simulink model "Drone_Model_Initial"  (R2024b)
settings: Solver=VariableStepAuto  StartTime=0.0  StopTime=22.5  MaxStep=1e-4  RelTol=1e-3
values from neighbouring files (symbols this model uses):
  Kd_angle = 2.6    [MainScript.m]
  Kd_angle_psi = 2.6    [MainScript.m]
  Kd_dist = 1.05    [MainScript.m]
  Kd_z = 4.4    [MainScript.m]
  Ki_angle = 0.5    [MainScript.m]
  Ki_angle_psi = 0.5    [MainScript.m]
  Ki_dist = 0    [MainScript.m]
  Ki_z = 0.1    [MainScript.m]
  Kp_angle = 2.95    [MainScript.m]
  Kp_angle_psi = 2.95    [MainScript.m]
  Kp_dist = 1    [MainScript.m]
  Kp_z = 2    [MainScript.m]
  p1 = (Iyy - Izz) / Ixx    [linearizeSystem.m]
  p3 = (Ixx - Iyy) / Iyy    [linearizeSystem.m]
  p4 = 1 / Iyy    [linearizeSystem.m]
  p6 = 1 / Izz    [linearizeSystem.m]
undefined symbols (not defined in the file or in its folder): g, K, m, Omega_sq_2_U, p7, phi_0, phi_dot_0, phi_limit, psi_0, psi_dot_0, th_0, th_dot_0, theta_limit, U_Sq_max, U_to_Omega_sq, x_0, x_dot_0, y_0, y_dot_0, z_0, z_dot_0
libraries: slpidlib x6, simulink x1
settings Model: Creator=jkord  LastModifiedBy=steli

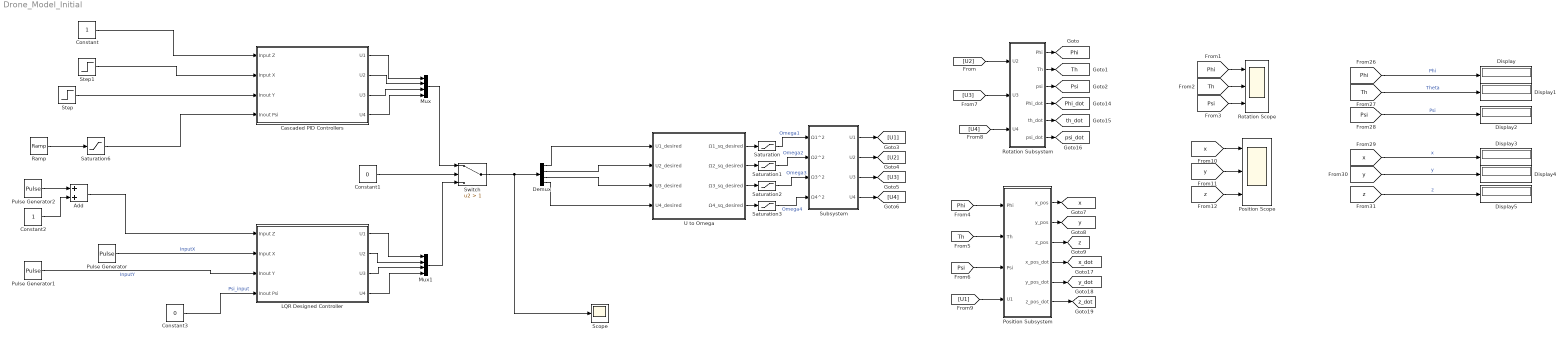
== system Drone_Model_Initial ==
  Add : Sum
  Cascaded PID Controllers : Subsystem
  Constant : Constant
  Constant1 : Constant  Value=0
  Constant2 : Constant
  Constant3 : Constant  Value=0
  Demux : Demux
  Display{,1..5} (6 alike) : Display
  LQR Designed Controller : Subsystem
  Mux : Mux
  Mux1 : Mux
  Position Subsystem : Subsystem
  Position Scope : Scope  NumInputPorts=3
  Pulse Generator : DiscretePulseGenerator  PulseType=Time based  Period=10  PulseWidth=50  PhaseDelay=2.5
  Pulse Generator1 : DiscretePulseGenerator  PulseType=Time based  Period=20  PulseWidth=50  PhaseDelay=10
  Pulse Generator2 : DiscretePulseGenerator  PulseType=Time based  Period=20  PulseWidth=50  PhaseDelay=5
  Ramp : simulink/Sources/Ramp  slope=0.01  start=2  InitialOutput=0
  Rotation Subsystem : Subsystem
  Rotation Scope : Scope  NumInputPorts=3
  Saturation{,1..3} (4 alike) : Saturate  UpperLimit=U_Sq_max  LowerLimit=0
  Saturation6 : Saturate  UpperLimit=0.2  LowerLimit=0
  Scope : Scope
  Step : Step  Time=5  SampleTime=0
  Step1 : Step  Time=2  SampleTime=0
  Subsystem : Subsystem
  Switch : Switch  Criteria=u2 > Threshold  Threshold=1  SaturateOnIntegerOverflow=off  InputSameDT=off
  U to Omega : Subsystem
  tag scope: Phi=global, Phi_dot=global, Psi=global, Th=global, psi_dot=global, th_dot=global, x=global, x_dot=global, y=global, y_dot=global, z=global, z_dot=global
  wires:
  [Th] -> Position Subsystem/2(Th)
  [U3] -> Rotation Subsystem/2(U3)
  Rotation Subsystem/3(psi) -> [Psi]
  [U4] -> Rotation Subsystem/3(U4)
  Rotation Subsystem/1(Phi) -> [Phi]
  Rotation Subsystem/2(Th) -> [Th]
  Position Subsystem/6(z_pos_dot) -> [z_dot]
  [Phi] -> Position Subsystem/1(Phi)
  Rotation Subsystem/4(Phi_dot) -> [Phi_dot]
  Rotation Subsystem/5(th_dot) -> [th_dot]
  Position Subsystem/4(x_pos_dot) -> [x_dot]
  [Psi] -> Position Subsystem/3(Psi)
  Position Subsystem/5(y_pos_dot) -> [y_dot]
  Position Subsystem/1(x_pos) -> [x]
  [U1] -> Position Subsystem/4(U1)
  Position Subsystem/3(z_pos) -> [z]
  Position Subsystem/2(y_pos) -> [y]
  [U2] -> Rotation Subsystem/1(U2)
  U to Omega/1(Ω1_sq_desired) -> Saturation/1
  Saturation3/1 -> Subsystem/4(Ω4^2)  "Omega4"
  U to Omega/3(Ω3_sq_desired) -> Saturation2/1
  U to Omega/2(Ω2_sq_desired) -> Saturation1/1
  Saturation2/1 -> Subsystem/3(Ω3^2)  "Omega3"
  Saturation1/1 -> Subsystem/2(Ω2^2)  "Omega2"
  U to Omega/4(Ω4_sq_desired) -> Saturation3/1
  Subsystem/4(U4) -> [U4]
  Saturation/1 -> Subsystem/1(Ω1^2)  "Omega1"
  Subsystem/2(U2) -> [U2]
  Subsystem/3(U3) -> [U3]
  Subsystem/1(U1) -> [U1]
  [Psi] -> Rotation Scope/3
  [z] -> Display5/1  "z"
  [Psi] -> Display2/1  "Psi"
  [Th] -> Rotation Scope/2
  [Th] -> Display1/1  "Theta"
  [y] -> Position Scope/2
  [Phi] -> Rotation Scope/1
  [z] -> Position Scope/3
  [Phi] -> Display/1  "Phi"
  [x] -> Display3/1  "x"
  [y] -> Display4/1  "y"
  [x] -> Position Scope/1
  Ramp/1 -> Saturation6/1
  Constant/1 -> Cascaded PID Controllers/1(Input Z)
  Step1/1 -> Cascaded PID Controllers/2(Input X)
  Step/1 -> Cascaded PID Controllers/3(Inout Y)
  Saturation6/1 -> Cascaded PID Controllers/4(Inout Psi)
  Cascaded PID Controllers/1(U1) -> Mux/1
  Cascaded PID Controllers/2(U2) -> Mux/2
  Cascaded PID Controllers/3(U3) -> Mux/3
  Cascaded PID Controllers/4(U4) -> Mux/4
  Mux/1 -> Switch/1
  Switch/1 -> Scope/1, Demux/1
  Demux/1 -> U to Omega/1(U1_desired)
  Demux/2 -> U to Omega/2(U2_desired)
  Demux/3 -> U to Omega/3(U3_desired)
  Demux/4 -> U to Omega/4(U4_desired)
  Constant1/1 -> Switch/2
  LQR Designed Controller/2(U2) -> Mux1/2
  LQR Designed Controller/1(U1) -> Mux1/1
  LQR Designed Controller/3(U3) -> Mux1/3
  LQR Designed Controller/4(U4) -> Mux1/4
  Mux1/1 -> Switch/3
  Rotation Subsystem/6(psi_dot) -> [psi_dot]
  Pulse Generator/1 -> LQR Designed Controller/2(Input X)  "InputX"
  Pulse Generator1/1 -> LQR Designed Controller/3(Inout Y)  "InputY"
  Pulse Generator2/1 -> Add/1
  Constant2/1 -> Add/2
  Add/1 -> LQR Designed Controller/1(Input Z)
  Constant3/1 -> LQR Designed Controller/4(Inout Psi)  "Psi_input"

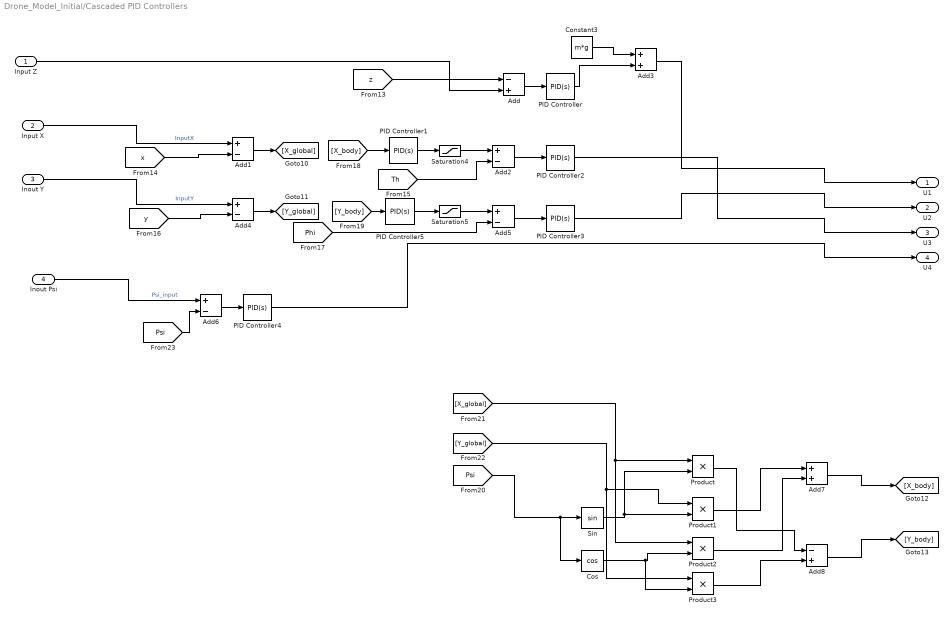
== system Drone_Model_Initial/Cascaded PID Controllers ==
  Input Z : Inport
  Input X : Inport  Port=2
  Inout Y : Inport  Port=3
  Inout Psi : Inport  Port=4
  Add : Sum  Inputs=-+
  Add{1..2,4..6} (5 alike) : Sum  Inputs=+-
  Add3 : Sum
  Add7 : Sum
  Add8 : Sum  Inputs=-+
  Constant3 : Constant  Value=m*g
  Cos : Trigonometry  Operator=cos
  PID Controller : slpidlib/PID Controller  Controller=PID  Form=Parallel  TimeDomain=Continuous-time  UseExternalTs=off  SampleTime=-1  IntegratorMethod=Forward Euler  FilterMethod=Forward Euler  ControllerParametersSource=internal  P=Kp_z  I=Ki_z  UseKiTs=off  D=Kd_z  UseExternalDerivativeSource=off  N=100  UseFilter=on  TunerSelectOption=Transfer Function Based (PID Tuner App)  InitialConditionSource=internal  InitialConditionForIntegrator=0  InitialConditionForFilter=0  DifferentiatorICPrevScaledInput=0  ExternalReset=none  TrackingMode=off  Kt=1  LimitOutput=off  SatLimitsSource=internal  UpperSaturationLimit=inf  LowerSaturationLimit=-inf  LinearizeAsGain=on  AntiWindupMode=none  Kb=1  LimitIntegrator=off  UpperIntegratorSaturationLimit=inf  LowerIntegratorSaturationLimit=-inf  POutMin=[]  POutMax=[]  IOutMin=[]  IOutMax=[]  DOutMin=[]  DOutMax=[]  NOutMin=[]  NOutMax=[]  SumOutMin=[]  SumOutMax=[]  SaturationOutMin=[]  SaturationOutMax=[]  PParamMin=[]  PParamMax=[]  IParamMin=[]  IParamMax=[]  DParamMin=[]  DParamMax=[]  NParamMin=[]  NParamMax=[]  KbParamMin=[]  KbParamMax=[]  KtParamMin=[]  KtParamMax=[]  KbOutMin=[]  KbOutMax=[]  KtOutMin=[]  KtOutMax=[]  IntegratorOutMin=[]  IntegratorOutMax=[]  FilterOutMin=[]  FilterOutMax=[]  SumI1OutMin=[]  SumI1OutMax=[]  SumI2OutMin=[]  SumI2OutMax=[]  SumI3OutMin=[]  SumI3OutMax=[]  SumI4OutMin=[]  SumI4OutMax=[]  SumDOutMin=[]  SumDOutMax=[]  DifferentiatorOutMin=[]  DifferentiatorOutMax=[]  FilterDiffOutCoefMin=[]  FilterDiffOutCoefMax=[]  ReciprocalOutMin=[]  ReciprocalOutMax=[]  SumDenOutMin=[]  SumDenOutMax=[]  SumNumOutMin=[]  SumNumOutMax=[]  DivideOutMin=[]  DivideOutMax=[]  UdiffTsProdOutMin=[]  UdiffTsProdOutMax=[]  NTsProdOutMin=[]  NTsProdOutMax=[]  UintegralTsProdOutMin=[]  UintegralTsProdOutMax=[]  UngainTsProdOutMin=[]  UngainTsProdOutMax=[]  ClampingZeroOutDataTypeStr=Inherit: Inherit via back propagation  ClampingZeroOutMin=[]  ClampingZeroOutMax=[]  FilterDenConstantOutDataTypeStr=Inherit: Inherit via back propagation  FilterDenConstantOutMin=[]  FilterDenConstantOutMax=[]  PCopyOutDataTypeStr=Inherit: Inherit via back propagation  PCopyOutMin=[]  PCopyOutMax=[]  NCopyOutDataTypeStr=Inherit: Inherit via back propagation  NCopyOutMin=[]  NCopyOutMax=[]  IntegratorContinuousStateAttributes=''  IntegratorStateMustResolveToSignalObject=off  IntegratorRTWStateStorageClass=Auto  FilterContinuousStateAttributes=''  FilterStateMustResolveToSignalObject=off  FilterRTWStateStorageClass=Auto  ParallelPVariant=InternalParameters  IdealPVariant=Disabled  IVariant=InternalParameters  DVariant=InternalParameters  IntegratorVariant=Continuous  SatVariant=Disabled  AWVariant=Passthrough  PCopyVariant=Disabled  TRVariant=Disabled  FdbkBlocksVariant=Forward  IdealPFdbkVariant=Disabled  SatFdbkVariant=Disabled  DerivativeFilterVariant=ContFilter  NVariant=InternalParameters  NCopyVariant=Disabled  FilterICVariant=InternalICsFilter  IntegratorICVariant=InternalICs  ExternalResetVariant=Disabled  TRSumVariant=Passthrough  SumFdbkVariant=Disabled  SumVariant=Sum_PID  TsampFilterVariant=InternalTs  TsampNgainVariant=Passthrough  TsampIntegralVariant=Disabled_SignalSpec  ExternalSaturationOutDataTypeStr=Inherit: Same as second input  DerivativeSourceVariant=ErrorSignal  PreIntVariant=InternalPreInt
  PID Controller1 : slpidlib/PID Controller  Controller=PID  Form=Parallel  TimeDomain=Continuous-time  UseExternalTs=off  SampleTime=-1  IntegratorMethod=Forward Euler  FilterMethod=Forward Euler  ControllerParametersSource=internal  P=Kp_dist  I=Ki_dist  UseKiTs=off  D=Kd_dist  UseExternalDerivativeSource=off  N=100  UseFilter=on  TunerSelectOption=Transfer Function Based (PID Tuner App)  InitialConditionSource=internal  InitialConditionForIntegrator=0  InitialConditionForFilter=0  DifferentiatorICPrevScaledInput=0  ExternalReset=none  TrackingMode=off  Kt=1  LimitOutput=off  SatLimitsSource=internal  UpperSaturationLimit=inf  LowerSaturationLimit=-inf  LinearizeAsGain=on  AntiWindupMode=none  Kb=1  LimitIntegrator=off  UpperIntegratorSaturationLimit=inf  LowerIntegratorSaturationLimit=-inf  POutMin=[]  POutMax=[]  IOutMin=[]  IOutMax=[]  DOutMin=[]  DOutMax=[]  NOutMin=[]  NOutMax=[]  SumOutMin=[]  SumOutMax=[]  SaturationOutMin=[]  SaturationOutMax=[]  PParamMin=[]  PParamMax=[]  IParamMin=[]  IParamMax=[]  DParamMin=[]  DParamMax=[]  NParamMin=[]  NParamMax=[]  KbParamMin=[]  KbParamMax=[]  KtParamMin=[]  KtParamMax=[]  KbOutMin=[]  KbOutMax=[]  KtOutMin=[]  KtOutMax=[]  IntegratorOutMin=[]  IntegratorOutMax=[]  FilterOutMin=[]  FilterOutMax=[]  SumI1OutMin=[]  SumI1OutMax=[]  SumI2OutMin=[]  SumI2OutMax=[]  SumI3OutMin=[]  SumI3OutMax=[]  SumI4OutMin=[]  SumI4OutMax=[]  SumDOutMin=[]  SumDOutMax=[]  DifferentiatorOutMin=[]  DifferentiatorOutMax=[]  FilterDiffOutCoefMin=[]  FilterDiffOutCoefMax=[]  ReciprocalOutMin=[]  ReciprocalOutMax=[]  SumDenOutMin=[]  SumDenOutMax=[]  SumNumOutMin=[]  SumNumOutMax=[]  DivideOutMin=[]  DivideOutMax=[]  UdiffTsProdOutMin=[]  UdiffTsProdOutMax=[]  NTsProdOutMin=[]  NTsProdOutMax=[]  UintegralTsProdOutMin=[]  UintegralTsProdOutMax=[]  UngainTsProdOutMin=[]  UngainTsProdOutMax=[]  ClampingZeroOutDataTypeStr=Inherit: Inherit via back propagation  ClampingZeroOutMin=[]  ClampingZeroOutMax=[]  FilterDenConstantOutDataTypeStr=Inherit: Inherit via back propagation  FilterDenConstantOutMin=[]  FilterDenConstantOutMax=[]  PCopyOutDataTypeStr=Inherit: Inherit via back propagation  PCopyOutMin=[]  PCopyOutMax=[]  NCopyOutDataTypeStr=Inherit: Inherit via back propagation  NCopyOutMin=[]  NCopyOutMax=[]  IntegratorContinuousStateAttributes=''  IntegratorStateMustResolveToSignalObject=off  IntegratorRTWStateStorageClass=Auto  FilterContinuousStateAttributes=''  FilterStateMustResolveToSignalObject=off  FilterRTWStateStorageClass=Auto  ParallelPVariant=InternalParameters  IdealPVariant=Disabled  IVariant=InternalParameters  DVariant=InternalParameters  IntegratorVariant=Continuous  SatVariant=Disabled  AWVariant=Passthrough  PCopyVariant=Disabled  TRVariant=Disabled  FdbkBlocksVariant=Forward  IdealPFdbkVariant=Disabled  SatFdbkVariant=Disabled  DerivativeFilterVariant=ContFilter  NVariant=InternalParameters  NCopyVariant=Disabled  FilterICVariant=InternalICsFilter  IntegratorICVariant=InternalICs  ExternalResetVariant=Disabled  TRSumVariant=Passthrough  SumFdbkVariant=Disabled  SumVariant=Sum_PID  TsampFilterVariant=InternalTs  TsampNgainVariant=Passthrough  TsampIntegralVariant=Disabled_SignalSpec  ExternalSaturationOutDataTypeStr=Inherit: Same as second input  DerivativeSourceVariant=ErrorSignal  PreIntVariant=InternalPreInt
  PID Controller2 : slpidlib/PID Controller  Controller=PID  Form=Parallel  TimeDomain=Continuous-time  UseExternalTs=off  SampleTime=-1  IntegratorMethod=Forward Euler  FilterMethod=Forward Euler  ControllerParametersSource=internal  P=Kp_angle  I=Ki_angle  UseKiTs=off  D=Kd_angle  UseExternalDerivativeSource=off  N=100  UseFilter=on  TunerSelectOption=Transfer Function Based (PID Tuner App)  InitialConditionSource=internal  InitialConditionForIntegrator=0  InitialConditionForFilter=0  DifferentiatorICPrevScaledInput=0  ExternalReset=none  TrackingMode=off  Kt=1  LimitOutput=off  SatLimitsSource=internal  UpperSaturationLimit=inf  LowerSaturationLimit=-inf  LinearizeAsGain=on  AntiWindupMode=none  Kb=1  LimitIntegrator=off  UpperIntegratorSaturationLimit=inf  LowerIntegratorSaturationLimit=-inf  POutMin=[]  POutMax=[]  IOutMin=[]  IOutMax=[]  DOutMin=[]  DOutMax=[]  NOutMin=[]  NOutMax=[]  SumOutMin=[]  SumOutMax=[]  SaturationOutMin=[]  SaturationOutMax=[]  PParamMin=[]  PParamMax=[]  IParamMin=[]  IParamMax=[]  DParamMin=[]  DParamMax=[]  NParamMin=[]  NParamMax=[]  KbParamMin=[]  KbParamMax=[]  KtParamMin=[]  KtParamMax=[]  KbOutMin=[]  KbOutMax=[]  KtOutMin=[]  KtOutMax=[]  IntegratorOutMin=[]  IntegratorOutMax=[]  FilterOutMin=[]  FilterOutMax=[]  SumI1OutMin=[]  SumI1OutMax=[]  SumI2OutMin=[]  SumI2OutMax=[]  SumI3OutMin=[]  SumI3OutMax=[]  SumI4OutMin=[]  SumI4OutMax=[]  SumDOutMin=[]  SumDOutMax=[]  DifferentiatorOutMin=[]  DifferentiatorOutMax=[]  FilterDiffOutCoefMin=[]  FilterDiffOutCoefMax=[]  ReciprocalOutMin=[]  ReciprocalOutMax=[]  SumDenOutMin=[]  SumDenOutMax=[]  SumNumOutMin=[]  SumNumOutMax=[]  DivideOutMin=[]  DivideOutMax=[]  UdiffTsProdOutMin=[]  UdiffTsProdOutMax=[]  NTsProdOutMin=[]  NTsProdOutMax=[]  UintegralTsProdOutMin=[]  UintegralTsProdOutMax=[]  UngainTsProdOutMin=[]  UngainTsProdOutMax=[]  ClampingZeroOutDataTypeStr=Inherit: Inherit via back propagation  ClampingZeroOutMin=[]  ClampingZeroOutMax=[]  FilterDenConstantOutDataTypeStr=Inherit: Inherit via back propagation  FilterDenConstantOutMin=[]  FilterDenConstantOutMax=[]  PCopyOutDataTypeStr=Inherit: Inherit via back propagation  PCopyOutMin=[]  PCopyOutMax=[]  NCopyOutDataTypeStr=Inherit: Inherit via back propagation  NCopyOutMin=[]  NCopyOutMax=[]  IntegratorContinuousStateAttributes=''  IntegratorStateMustResolveToSignalObject=off  IntegratorRTWStateStorageClass=Auto  FilterContinuousStateAttributes=''  FilterStateMustResolveToSignalObject=off  FilterRTWStateStorageClass=Auto  ParallelPVariant=InternalParameters  IdealPVariant=Disabled  IVariant=InternalParameters  DVariant=InternalParameters  IntegratorVariant=Continuous  SatVariant=Disabled  AWVariant=Passthrough  PCopyVariant=Disabled  TRVariant=Disabled  FdbkBlocksVariant=Forward  IdealPFdbkVariant=Disabled  SatFdbkVariant=Disabled  DerivativeFilterVariant=ContFilter  NVariant=InternalParameters  NCopyVariant=Disabled  FilterICVariant=InternalICsFilter  IntegratorICVariant=InternalICs  ExternalResetVariant=Disabled  TRSumVariant=Passthrough  SumFdbkVariant=Disabled  SumVariant=Sum_PID  TsampFilterVariant=InternalTs  TsampNgainVariant=Passthrough  TsampIntegralVariant=Disabled_SignalSpec  ExternalSaturationOutDataTypeStr=Inherit: Same as second input  DerivativeSourceVariant=ErrorSignal  PreIntVariant=InternalPreInt
  PID Controller3 : slpidlib/PID Controller  Controller=PID  Form=Parallel  TimeDomain=Continuous-time  UseExternalTs=off  SampleTime=-1  IntegratorMethod=Forward Euler  FilterMethod=Forward Euler  ControllerParametersSource=internal  P=Kp_angle  I=Ki_angle  UseKiTs=off  D=Kd_angle  UseExternalDerivativeSource=off  N=100  UseFilter=on  TunerSelectOption=Transfer Function Based (PID Tuner App)  InitialConditionSource=internal  InitialConditionForIntegrator=0  InitialConditionForFilter=0  DifferentiatorICPrevScaledInput=0  ExternalReset=none  TrackingMode=off  Kt=1  LimitOutput=off  SatLimitsSource=internal  UpperSaturationLimit=inf  LowerSaturationLimit=-inf  LinearizeAsGain=on  AntiWindupMode=none  Kb=1  LimitIntegrator=off  UpperIntegratorSaturationLimit=inf  LowerIntegratorSaturationLimit=-inf  POutMin=[]  POutMax=[]  IOutMin=[]  IOutMax=[]  DOutMin=[]  DOutMax=[]  NOutMin=[]  NOutMax=[]  SumOutMin=[]  SumOutMax=[]  SaturationOutMin=[]  SaturationOutMax=[]  PParamMin=[]  PParamMax=[]  IParamMin=[]  IParamMax=[]  DParamMin=[]  DParamMax=[]  NParamMin=[]  NParamMax=[]  KbParamMin=[]  KbParamMax=[]  KtParamMin=[]  KtParamMax=[]  KbOutMin=[]  KbOutMax=[]  KtOutMin=[]  KtOutMax=[]  IntegratorOutMin=[]  IntegratorOutMax=[]  FilterOutMin=[]  FilterOutMax=[]  SumI1OutMin=[]  SumI1OutMax=[]  SumI2OutMin=[]  SumI2OutMax=[]  SumI3OutMin=[]  SumI3OutMax=[]  SumI4OutMin=[]  SumI4OutMax=[]  SumDOutMin=[]  SumDOutMax=[]  DifferentiatorOutMin=[]  DifferentiatorOutMax=[]  FilterDiffOutCoefMin=[]  FilterDiffOutCoefMax=[]  ReciprocalOutMin=[]  ReciprocalOutMax=[]  SumDenOutMin=[]  SumDenOutMax=[]  SumNumOutMin=[]  SumNumOutMax=[]  DivideOutMin=[]  DivideOutMax=[]  UdiffTsProdOutMin=[]  UdiffTsProdOutMax=[]  NTsProdOutMin=[]  NTsProdOutMax=[]  UintegralTsProdOutMin=[]  UintegralTsProdOutMax=[]  UngainTsProdOutMin=[]  UngainTsProdOutMax=[]  ClampingZeroOutDataTypeStr=Inherit: Inherit via back propagation  ClampingZeroOutMin=[]  ClampingZeroOutMax=[]  FilterDenConstantOutDataTypeStr=Inherit: Inherit via back propagation  FilterDenConstantOutMin=[]  FilterDenConstantOutMax=[]  PCopyOutDataTypeStr=Inherit: Inherit via back propagation  PCopyOutMin=[]  PCopyOutMax=[]  NCopyOutDataTypeStr=Inherit: Inherit via back propagation  NCopyOutMin=[]  NCopyOutMax=[]  IntegratorContinuousStateAttributes=''  IntegratorStateMustResolveToSignalObject=off  IntegratorRTWStateStorageClass=Auto  FilterContinuousStateAttributes=''  FilterStateMustResolveToSignalObject=off  FilterRTWStateStorageClass=Auto  ParallelPVariant=InternalParameters  IdealPVariant=Disabled  IVariant=InternalParameters  DVariant=InternalParameters  IntegratorVariant=Continuous  SatVariant=Disabled  AWVariant=Passthrough  PCopyVariant=Disabled  TRVariant=Disabled  FdbkBlocksVariant=Forward  IdealPFdbkVariant=Disabled  SatFdbkVariant=Disabled  DerivativeFilterVariant=ContFilter  NVariant=InternalParameters  NCopyVariant=Disabled  FilterICVariant=InternalICsFilter  IntegratorICVariant=InternalICs  ExternalResetVariant=Disabled  TRSumVariant=Passthrough  SumFdbkVariant=Disabled  SumVariant=Sum_PID  TsampFilterVariant=InternalTs  TsampNgainVariant=Passthrough  TsampIntegralVariant=Disabled_SignalSpec  ExternalSaturationOutDataTypeStr=Inherit: Same as second input  DerivativeSourceVariant=ErrorSignal  PreIntVariant=InternalPreInt
  PID Controller4 : slpidlib/PID Controller  Controller=PID  Form=Parallel  TimeDomain=Continuous-time  UseExternalTs=off  SampleTime=-1  IntegratorMethod=Forward Euler  FilterMethod=Forward Euler  ControllerParametersSource=internal  P=Kp_angle_psi  I=Ki_angle_psi  UseKiTs=off  D=Kd_angle_psi  UseExternalDerivativeSource=off  N=100  UseFilter=on  TunerSelectOption=Transfer Function Based (PID Tuner App)  InitialConditionSource=internal  InitialConditionForIntegrator=0  InitialConditionForFilter=0  DifferentiatorICPrevScaledInput=0  ExternalReset=none  TrackingMode=off  Kt=1  LimitOutput=off  SatLimitsSource=internal  UpperSaturationLimit=inf  LowerSaturationLimit=-inf  LinearizeAsGain=on  AntiWindupMode=none  Kb=1  LimitIntegrator=off  UpperIntegratorSaturationLimit=inf  LowerIntegratorSaturationLimit=-inf  POutMin=[]  POutMax=[]  IOutMin=[]  IOutMax=[]  DOutMin=[]  DOutMax=[]  NOutMin=[]  NOutMax=[]  SumOutMin=[]  SumOutMax=[]  SaturationOutMin=[]  SaturationOutMax=[]  PParamMin=[]  PParamMax=[]  IParamMin=[]  IParamMax=[]  DParamMin=[]  DParamMax=[]  NParamMin=[]  NParamMax=[]  KbParamMin=[]  KbParamMax=[]  KtParamMin=[]  KtParamMax=[]  KbOutMin=[]  KbOutMax=[]  KtOutMin=[]  KtOutMax=[]  IntegratorOutMin=[]  IntegratorOutMax=[]  FilterOutMin=[]  FilterOutMax=[]  SumI1OutMin=[]  SumI1OutMax=[]  SumI2OutMin=[]  SumI2OutMax=[]  SumI3OutMin=[]  SumI3OutMax=[]  SumI4OutMin=[]  SumI4OutMax=[]  SumDOutMin=[]  SumDOutMax=[]  DifferentiatorOutMin=[]  DifferentiatorOutMax=[]  FilterDiffOutCoefMin=[]  FilterDiffOutCoefMax=[]  ReciprocalOutMin=[]  ReciprocalOutMax=[]  SumDenOutMin=[]  SumDenOutMax=[]  SumNumOutMin=[]  SumNumOutMax=[]  DivideOutMin=[]  DivideOutMax=[]  UdiffTsProdOutMin=[]  UdiffTsProdOutMax=[]  NTsProdOutMin=[]  NTsProdOutMax=[]  UintegralTsProdOutMin=[]  UintegralTsProdOutMax=[]  UngainTsProdOutMin=[]  UngainTsProdOutMax=[]  ClampingZeroOutDataTypeStr=Inherit: Inherit via back propagation  ClampingZeroOutMin=[]  ClampingZeroOutMax=[]  FilterDenConstantOutDataTypeStr=Inherit: Inherit via back propagation  FilterDenConstantOutMin=[]  FilterDenConstantOutMax=[]  PCopyOutDataTypeStr=Inherit: Inherit via back propagation  PCopyOutMin=[]  PCopyOutMax=[]  NCopyOutDataTypeStr=Inherit: Inherit via back propagation  NCopyOutMin=[]  NCopyOutMax=[]  IntegratorContinuousStateAttributes=''  IntegratorStateMustResolveToSignalObject=off  IntegratorRTWStateStorageClass=Auto  FilterContinuousStateAttributes=''  FilterStateMustResolveToSignalObject=off  FilterRTWStateStorageClass=Auto  ParallelPVariant=InternalParameters  IdealPVariant=Disabled  IVariant=InternalParameters  DVariant=InternalParameters  IntegratorVariant=Continuous  SatVariant=Disabled  AWVariant=Passthrough  PCopyVariant=Disabled  TRVariant=Disabled  FdbkBlocksVariant=Forward  IdealPFdbkVariant=Disabled  SatFdbkVariant=Disabled  DerivativeFilterVariant=ContFilter  NVariant=InternalParameters  NCopyVariant=Disabled  FilterICVariant=InternalICsFilter  IntegratorICVariant=InternalICs  ExternalResetVariant=Disabled  TRSumVariant=Passthrough  SumFdbkVariant=Disabled  SumVariant=Sum_PID  TsampFilterVariant=InternalTs  TsampNgainVariant=Passthrough  TsampIntegralVariant=Disabled_SignalSpec  ExternalSaturationOutDataTypeStr=Inherit: Same as second input  DerivativeSourceVariant=ErrorSignal  PreIntVariant=InternalPreInt
  PID Controller5 : slpidlib/PID Controller  Controller=PID  Form=Parallel  TimeDomain=Continuous-time  UseExternalTs=off  SampleTime=-1  IntegratorMethod=Forward Euler  FilterMethod=Forward Euler  ControllerParametersSource=internal  P=Kp_dist  I=Ki_dist  UseKiTs=off  D=Kd_dist  UseExternalDerivativeSource=off  N=100  UseFilter=on  TunerSelectOption=Transfer Function Based (PID Tuner App)  InitialConditionSource=internal  InitialConditionForIntegrator=0  InitialConditionForFilter=0  DifferentiatorICPrevScaledInput=0  ExternalReset=none  TrackingMode=off  Kt=1  LimitOutput=off  SatLimitsSource=internal  UpperSaturationLimit=inf  LowerSaturationLimit=-inf  LinearizeAsGain=on  AntiWindupMode=none  Kb=1  LimitIntegrator=off  UpperIntegratorSaturationLimit=inf  LowerIntegratorSaturationLimit=-inf  POutMin=[]  POutMax=[]  IOutMin=[]  IOutMax=[]  DOutMin=[]  DOutMax=[]  NOutMin=[]  NOutMax=[]  SumOutMin=[]  SumOutMax=[]  SaturationOutMin=[]  SaturationOutMax=[]  PParamMin=[]  PParamMax=[]  IParamMin=[]  IParamMax=[]  DParamMin=[]  DParamMax=[]  NParamMin=[]  NParamMax=[]  KbParamMin=[]  KbParamMax=[]  KtParamMin=[]  KtParamMax=[]  KbOutMin=[]  KbOutMax=[]  KtOutMin=[]  KtOutMax=[]  IntegratorOutMin=[]  IntegratorOutMax=[]  FilterOutMin=[]  FilterOutMax=[]  SumI1OutMin=[]  SumI1OutMax=[]  SumI2OutMin=[]  SumI2OutMax=[]  SumI3OutMin=[]  SumI3OutMax=[]  SumI4OutMin=[]  SumI4OutMax=[]  SumDOutMin=[]  SumDOutMax=[]  DifferentiatorOutMin=[]  DifferentiatorOutMax=[]  FilterDiffOutCoefMin=[]  FilterDiffOutCoefMax=[]  ReciprocalOutMin=[]  ReciprocalOutMax=[]  SumDenOutMin=[]  SumDenOutMax=[]  SumNumOutMin=[]  SumNumOutMax=[]  DivideOutMin=[]  DivideOutMax=[]  UdiffTsProdOutMin=[]  UdiffTsProdOutMax=[]  NTsProdOutMin=[]  NTsProdOutMax=[]  UintegralTsProdOutMin=[]  UintegralTsProdOutMax=[]  UngainTsProdOutMin=[]  UngainTsProdOutMax=[]  ClampingZeroOutDataTypeStr=Inherit: Inherit via back propagation  ClampingZeroOutMin=[]  ClampingZeroOutMax=[]  FilterDenConstantOutDataTypeStr=Inherit: Inherit via back propagation  FilterDenConstantOutMin=[]  FilterDenConstantOutMax=[]  PCopyOutDataTypeStr=Inherit: Inherit via back propagation  PCopyOutMin=[]  PCopyOutMax=[]  NCopyOutDataTypeStr=Inherit: Inherit via back propagation  NCopyOutMin=[]  NCopyOutMax=[]  IntegratorContinuousStateAttributes=''  IntegratorStateMustResolveToSignalObject=off  IntegratorRTWStateStorageClass=Auto  FilterContinuousStateAttributes=''  FilterStateMustResolveToSignalObject=off  FilterRTWStateStorageClass=Auto  ParallelPVariant=InternalParameters  IdealPVariant=Disabled  IVariant=InternalParameters  DVariant=InternalParameters  IntegratorVariant=Continuous  SatVariant=Disabled  AWVariant=Passthrough  PCopyVariant=Disabled  TRVariant=Disabled  FdbkBlocksVariant=Forward  IdealPFdbkVariant=Disabled  SatFdbkVariant=Disabled  DerivativeFilterVariant=ContFilter  NVariant=InternalParameters  NCopyVariant=Disabled  FilterICVariant=InternalICsFilter  IntegratorICVariant=InternalICs  ExternalResetVariant=Disabled  TRSumVariant=Passthrough  SumFdbkVariant=Disabled  SumVariant=Sum_PID  TsampFilterVariant=InternalTs  TsampNgainVariant=Passthrough  TsampIntegralVariant=Disabled_SignalSpec  ExternalSaturationOutDataTypeStr=Inherit: Same as second input  DerivativeSourceVariant=ErrorSignal  PreIntVariant=InternalPreInt
  Product{,1..3} (4 alike) : Product
  Saturation4 : Saturate  UpperLimit=theta_limit  LowerLimit=-theta_limit
  Saturation5 : Saturate  UpperLimit=phi_limit  LowerLimit=-phi_limit
  Sin : Trigonometry
  U1 : Outport
  U2 : Outport  Port=2
  U3 : Outport  Port=3
  U4 : Outport  Port=4
  wires:
  PID Controller3/1 -> U2/1
  [y] -> Add4/2
  PID Controller1/1 -> Saturation4/1
  Constant3/1 -> Add3/1
  Add4/1 -> [Y_global]
  Add5/1 -> PID Controller3/1
  Add2/1 -> PID Controller2/1
  [Y_body] -> PID Controller5/1
  [x] -> Add1/2
  Saturation4/1 -> Add2/1
  [Psi] -> Add6/2
  Input X/1 -> Add1/1  "InputX"
  Inout Psi/1 -> Add6/1  "Psi_input"
  Add3/1 -> U1/1
  PID Controller/1 -> Add3/2
  [Phi] -> Add5/2
  Inout Y/1 -> Add4/1  "InputY"
  Add/1 -> PID Controller/1
  Saturation5/1 -> Add5/1
  PID Controller5/1 -> Saturation5/1
  Input Z/1 -> Add/2
  [z] -> Add/1
  [X_body] -> PID Controller1/1
  PID Controller2/1 -> U3/1
  Add1/1 -> [X_global]
  [Th] -> Add2/2
  PID Controller4/1 -> U4/1
  Add6/1 -> PID Controller4/1
  Product2/1 -> Add7/2
  [Y_global] -> Product3/1, Product1/1
  Product/1 -> Add8/1
  Sin/1 -> Product1/2, Product/2
  Add7/1 -> [X_body]
  Add8/1 -> [Y_body]
  [Psi] -> Cos/1, Sin/1
  [X_global] -> Product2/1, Product/1
  Product3/1 -> Add8/2
  Cos/1 -> Product3/2, Product2/2
  Product1/1 -> Add7/1

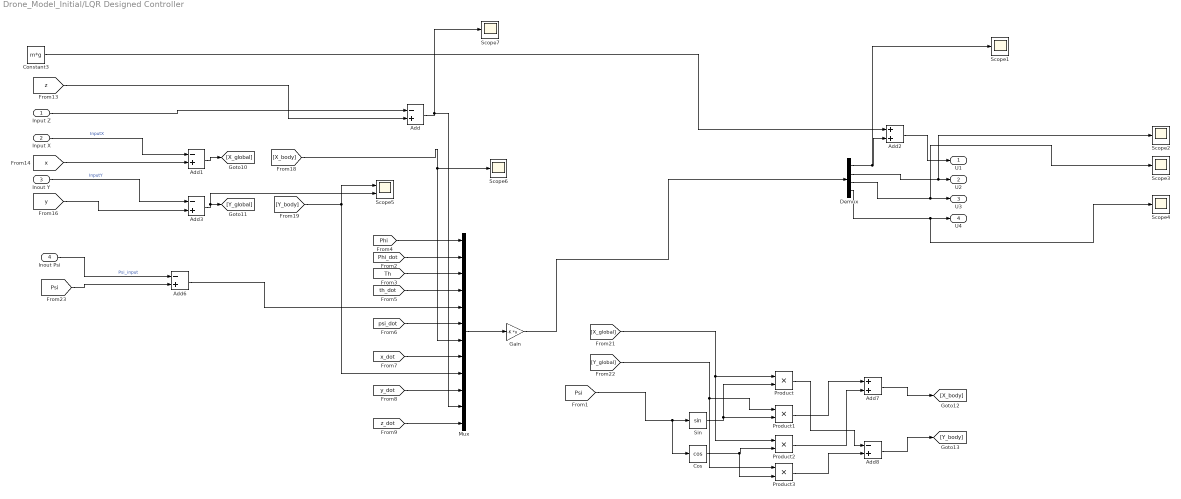
== system Drone_Model_Initial/LQR Designed Controller ==
  Input Z : Inport
  Input X : Inport  Port=2
  Inout Y : Inport  Port=3
  Inout Psi : Inport  Port=4
  Add{,1,3,6,8} (5 alike) : Sum  Inputs=-+
  Add2 : Sum
  Add7 : Sum
  Constant3 : Constant  Value=m*g
  Cos : Trigonometry  Operator=cos
  Demux : Demux
  Gain : Gain  Gain=-K  Multiplication=Matrix(K*u)
  Mux : Mux  Inputs=12
  Product{,1..3} (4 alike) : Product
  Scope{1..4,6..7} (6 alike) : Scope
  Scope5 : Scope  NumInputPorts=2
  Sin : Trigonometry
  U1 : Outport
  U2 : Outport  Port=2
  U3 : Outport  Port=3
  U4 : Outport  Port=4
  wires:
  [y] -> Add3/2
  Constant3/1 -> Add2/1
  Add3/1 -> Scope5/2, [Y_global]
  [x] -> Add1/2
  [Psi] -> Add6/2
  Input X/1 -> Add1/1  "InputX"
  Inout Psi/1 -> Add6/1  "Psi_input"
  Inout Y/1 -> Add3/1  "InputY"
  Input Z/1 -> Add/1
  [z] -> Add/2
  Add1/1 -> [X_global]
  Product2/1 -> Add7/2
  [Y_global] -> Product3/1, Product1/1
  Product/1 -> Add8/1
  Sin/1 -> Product1/2, Product/2
  Add7/1 -> [X_body]
  Add8/1 -> [Y_body]
  [X_global] -> Product2/1, Product/1
  Product3/1 -> Add8/2
  Cos/1 -> Product3/2, Product2/2
  Product1/1 -> Add7/1
  Gain/1 -> Demux/1
  Mux/1 -> Gain/1
  Add/1 -> Scope7/1, Mux/11
  [X_body] -> Mux/7, Scope6/1
  [Y_body] -> Scope5/1, Mux/9
  Add6/1 -> Mux/5
  [Phi] -> Mux/1
  Demux/1 -> Scope1/1, Add2/2
  Add2/1 -> U1/1
  [Phi_dot] -> Mux/2
  [Th] -> Mux/3
  [th_dot] -> Mux/4
  [psi_dot] -> Mux/6
  [x_dot] -> Mux/8
  [y_dot] -> Mux/10
  [z_dot] -> Mux/12
  Demux/4 -> Scope4/1, U4/1
  Demux/2 -> Scope2/1, U2/1
  Demux/3 -> Scope3/1, U3/1
  [Psi] -> Cos/1, Sin/1

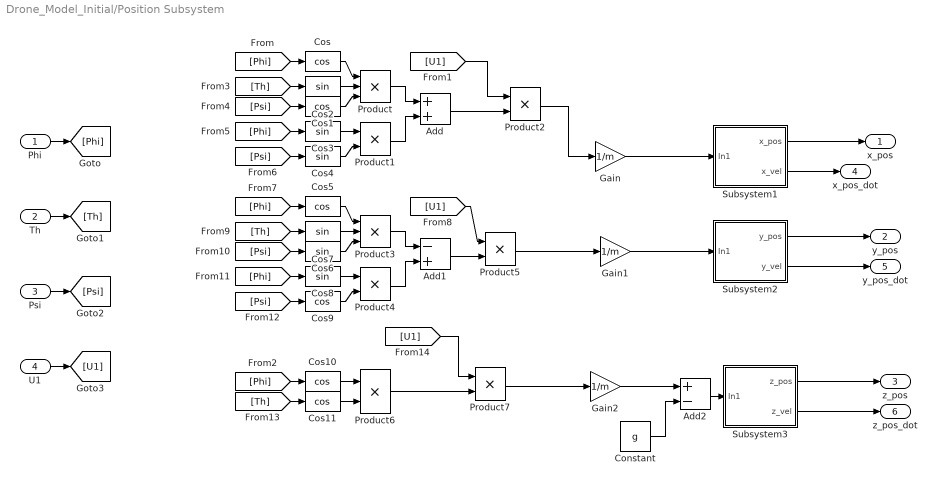
== system Drone_Model_Initial/Position Subsystem ==
  Phi : Inport
  Th : Inport  Port=2
  Psi : Inport  Port=3
  U1 : Inport  Port=4
  Add : Sum
  Add1 : Sum  Inputs=-+
  Add2 : Sum  Inputs=+-
  Constant : Constant  Value=g
  Cos{,1,5,9..11} (6 alike) : Trigonometry  Operator=cos
  Cos{2..4,6..8} (6 alike) : Trigonometry
  Gain : Gain  Gain=1/m
  Gain1 : Gain  Gain=1/m
  Gain2 : Gain  Gain=1/m
  Product : Product  Inputs=3
  Product{1..2,4..7} (6 alike) : Product
  Product3 : Product  Inputs=3
  Subsystem1 : Subsystem
  Subsystem2 : Subsystem
  Subsystem3 : Subsystem
  x_pos : Outport
  y_pos : Outport  Port=2
  z_pos : Outport  Port=3
  x_pos_dot : Outport  Port=4
  y_pos_dot : Outport  Port=5
  z_pos_dot : Outport  Port=6
  wires:
  Subsystem3/1(z_pos) -> z_pos/1
  Subsystem3/2(z_vel) -> z_pos_dot/1
  Subsystem1/1(x_pos) -> x_pos/1
  Subsystem2/1(y_pos) -> y_pos/1
  Subsystem2/2(y_vel) -> y_pos_dot/1
  Phi/1 -> [Phi]
  Th/1 -> [Th]
  Psi/1 -> [Psi]
  [Phi] -> Cos/1
  [Psi] -> Cos1/1
  [Th] -> Cos2/1
  Cos2/1 -> Product/2
  Cos/1 -> Product/1
  Cos1/1 -> Product/3
  Product/1 -> Add/1
  [Phi] -> Cos3/1
  [Psi] -> Cos4/1
  Cos3/1 -> Product1/1
  Cos4/1 -> Product1/2
  Product1/1 -> Add/2
  U1/1 -> [U1]
  [U1] -> Product2/1
  Add/1 -> Product2/2
  Product2/1 -> Gain/1
  Gain/1 -> Subsystem1/1(In1)
  [Phi] -> Cos5/1
  [Psi] -> Cos6/1
  [Phi] -> Cos8/1
  Cos6/1 -> Product3/3
  Add1/1 -> Product5/2
  Gain1/1 -> Subsystem2/1(In1)
  [Psi] -> Cos9/1
  Product4/1 -> Add1/2
  [U1] -> Product5/1
  Product3/1 -> Add1/1
  Cos5/1 -> Product3/1
  Cos7/1 -> Product3/2
  Cos9/1 -> Product4/2
  Cos8/1 -> Product4/1
  [Th] -> Cos7/1
  Product5/1 -> Gain1/1
  Add2/1 -> Subsystem3/1(In1)
  [Phi] -> Cos10/1
  Cos10/1 -> Product6/1
  Cos11/1 -> Product6/2
  [Th] -> Cos11/1
  [U1] -> Product7/1
  Product6/1 -> Product7/2
  Gain2/1 -> Add2/1
  Product7/1 -> Gain2/1
  Constant/1 -> Add2/2
  Subsystem1/2(x_vel) -> x_pos_dot/1

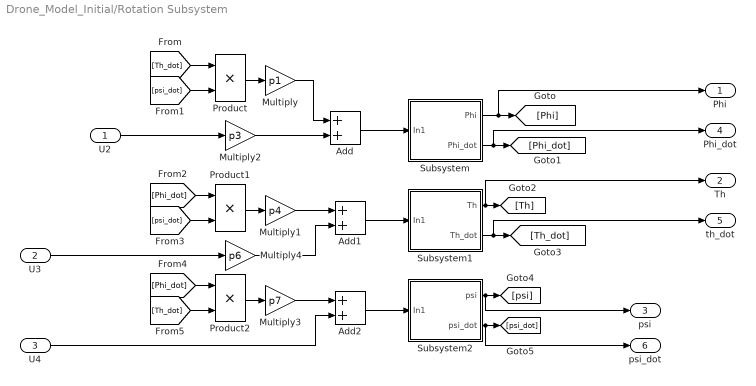
== system Drone_Model_Initial/Rotation Subsystem ==
  U2 : Inport
  U3 : Inport  Port=2
  U4 : Inport  Port=3
  Add : Sum
  Add1 : Sum
  Add2 : Sum
  Multiply : Gain  Gain=p1
  Multiply1 : Gain  Gain=p4
  Multiply2 : Gain  Gain=p3
  Multiply3 : Gain  Gain=p7
  Multiply4 : Gain  Gain=p6
  Product : Product
  Product1 : Product
  Product2 : Product
  Subsystem : Subsystem
  Subsystem1 : Subsystem
  Subsystem2 : Subsystem
  Phi : Outport
  Th : Outport  Port=2
  psi : Outport  Port=3
  Phi_dot : Outport  Port=4
  th_dot : Outport  Port=5
  psi_dot : Outport  Port=6
  wires:
  Subsystem2/1(psi) -> psi/1, [psi]
  [psi_dot] -> Product1/2
  Subsystem2/2(psi_dot) -> psi_dot/1, [psi_dot]
  Multiply2/1 -> Add/2
  Subsystem/2(Phi_dot) -> Phi_dot/1, [Phi_dot]
  Subsystem/1(Phi) -> Phi/1, [Phi]
  Product/1 -> Multiply/1
  Subsystem1/1(Th) -> Th/1, [Th]
  Product1/1 -> Multiply1/1
  [Phi_dot] -> Product1/1
  Multiply/1 -> Add/1
  Add/1 -> Subsystem/1(In1)
  [Th_dot] -> Product2/2
  Add2/1 -> Subsystem2/1(In1)
  Multiply1/1 -> Add1/1
  [psi_dot] -> Product/2
  Subsystem1/2(Th_dot) -> th_dot/1, [Th_dot]
  Multiply3/1 -> Add2/1
  [Th_dot] -> Product/1
  Add1/1 -> Subsystem1/1(In1)
  [Phi_dot] -> Product2/1
  Product2/1 -> Multiply3/1
  U3/1 -> Multiply4/1
  U2/1 -> Multiply2/1
  U4/1 -> Add2/2
  Multiply4/1 -> Add1/2

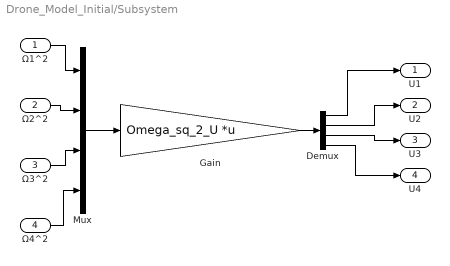
== system Drone_Model_Initial/Subsystem ==
  Ω1^2 : Inport
  Ω2^2 : Inport  Port=2
  Ω3^2 : Inport  Port=3
  Ω4^2 : Inport  Port=4
  Demux : Demux
  Gain : Gain  Gain=Omega_sq_2_U  Multiplication=Matrix(K*u)
  Mux : Mux
  U1 : Outport
  U2 : Outport  Port=2
  U3 : Outport  Port=3
  U4 : Outport  Port=4
  wires:
  Ω2^2/1 -> Mux/2
  Ω3^2/1 -> Mux/3
  Ω1^2/1 -> Mux/1
  Ω4^2/1 -> Mux/4
  Mux/1 -> Gain/1
  Gain/1 -> Demux/1
  Demux/1 -> U1/1
  Demux/2 -> U2/1
  Demux/3 -> U3/1
  Demux/4 -> U4/1

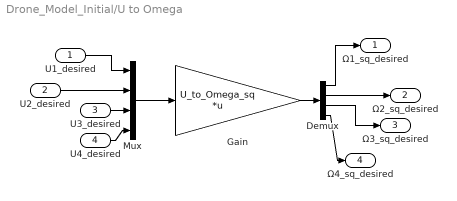
== system Drone_Model_Initial/U to Omega ==
  U1_desired : Inport
  U2_desired : Inport  Port=2
  U3_desired : Inport  Port=3
  U4_desired : Inport  Port=4
  Demux : Demux
  Gain : Gain  Gain=U_to_Omega_sq  Multiplication=Matrix(K*u)
  Mux : Mux
  Ω1_sq_desired : Outport
  Ω2_sq_desired : Outport  Port=2
  Ω3_sq_desired : Outport  Port=3
  Ω4_sq_desired : Outport  Port=4
  wires:
  U4_desired/1 -> Mux/4
  U1_desired/1 -> Mux/1
  Demux/3 -> Ω3_sq_desired/1
  Mux/1 -> Gain/1
  Demux/2 -> Ω2_sq_desired/1
  U2_desired/1 -> Mux/2
  Demux/4 -> Ω4_sq_desired/1
  U3_desired/1 -> Mux/3
  Demux/1 -> Ω1_sq_desired/1
  Gain/1 -> Demux/1

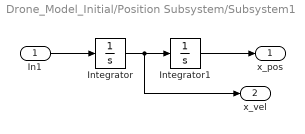
== system Drone_Model_Initial/Position Subsystem/Subsystem1 ==
  In1 : Inport
  Integrator : Integrator  InitialCondition=x_dot_0
  Integrator1 : Integrator  InitialCondition=x_0
  x_pos : Outport
  x_vel : Outport  Port=2
  wires:
  Integrator/1 -> x_vel/1, Integrator1/1
  In1/1 -> Integrator/1
  Integrator1/1 -> x_pos/1

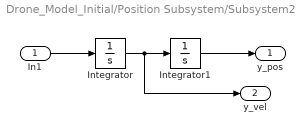
== system Drone_Model_Initial/Position Subsystem/Subsystem2 ==
  In1 : Inport
  Integrator : Integrator  InitialCondition=y_dot_0
  Integrator1 : Integrator  InitialCondition=y_0
  y_pos : Outport
  y_vel : Outport  Port=2
  wires:
  Integrator1/1 -> y_pos/1
  In1/1 -> Integrator/1
  Integrator/1 -> Integrator1/1, y_vel/1

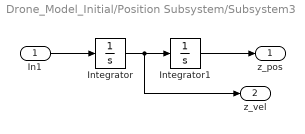
== system Drone_Model_Initial/Position Subsystem/Subsystem3 ==
  In1 : Inport
  Integrator : Integrator  InitialCondition=z_dot_0
  Integrator1 : Integrator  InitialCondition=z_0
  z_pos : Outport
  z_vel : Outport  Port=2
  wires:
  Integrator/1 -> z_vel/1, Integrator1/1
  In1/1 -> Integrator/1
  Integrator1/1 -> z_pos/1

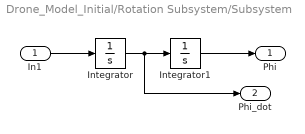
== system Drone_Model_Initial/Rotation Subsystem/Subsystem ==
  In1 : Inport
  Integrator : Integrator  InitialCondition=phi_dot_0
  Integrator1 : Integrator  InitialCondition=phi_0
  Phi : Outport
  Phi_dot : Outport  Port=2
  wires:
  Integrator/1 -> Phi_dot/1, Integrator1/1
  In1/1 -> Integrator/1
  Integrator1/1 -> Phi/1

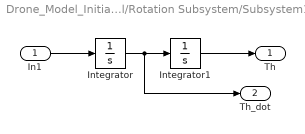
== system Drone_Model_Initial/Rotation Subsystem/Subsystem1 ==
  In1 : Inport
  Integrator : Integrator  InitialCondition=th_dot_0
  Integrator1 : Integrator  InitialCondition=th_0
  Th : Outport
  Th_dot : Outport  Port=2
  wires:
  Integrator1/1 -> Th/1
  In1/1 -> Integrator/1
  Integrator/1 -> Integrator1/1, Th_dot/1

== system Drone_Model_Initial/Rotation Subsystem/Subsystem2 ==
  In1 : Inport
  Integrator : Integrator  InitialCondition=psi_dot_0
  Integrator1 : Integrator  InitialCondition=psi_0
  psi : Outport
  psi_dot : Outport  Port=2
  wires:
  Integrator/1 -> psi_dot/1, Integrator1/1
  In1/1 -> Integrator/1
  Integrator1/1 -> psi/1
